simulink library "cooling_system_components"  (R2026a)
settings: Solver=VariableStepAuto
undefined symbols (not defined in the file or in its folder): cooling_system, plate_5p48s_detailled_thr
libraries: fl_lib x14, batt_lib x3, simulink x1, nesl_utility x1
Description:
  | Copyright 2023-2026 The MathWorks, Inc.
settings Model: Creator=smiller  LastModifiedBy=smiller

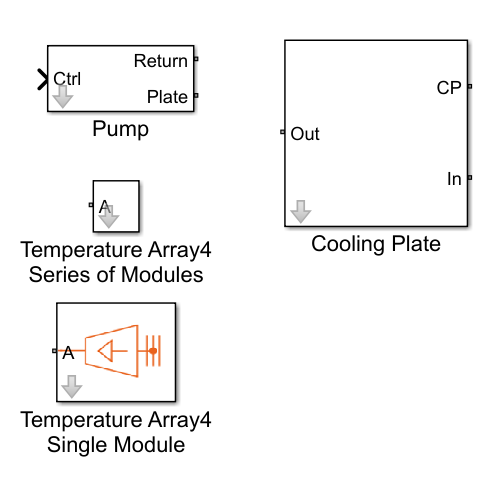
[thumbnail: Simulink's stored preview of the top-level diagram]
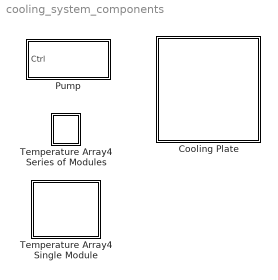
== system cooling_system_components ==
  Cooling Plate : Subsystem  mask{plate=plate_5p48s_detailled_thr}
      mask prompts: plate "Plate Parameters"
  Pump : Subsystem  mask{num_plates=8}
      mask prompts: num_plates "Number of plates"
  Temperature Array4 Series of Modules : Subsystem  mask{ma_num=1, ma_total=8, t_in=16, t_out=23}
      mask prompts: ma_num "Module Assembly Number"; ma_total "Total Module Assemblies"; t_in "Temperature System Inlet (degC)"; t_out "Temperature System Outlet (degC)"
  Temperature Array4 Single Module : Subsystem  mask{t_in=16, t_out=23}
      mask prompts: t_in "Temperature System Inlet (degC)"; t_out "Temperature System Outlet (degC)"
      mask Display: image('ssc_airvtol_cooling_bcs_IMAGE.png');

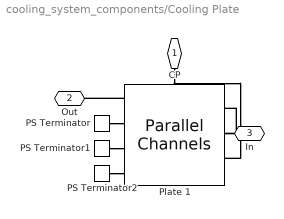
== system cooling_system_components/Cooling Plate ==
  PS Terminator : fl_lib/Physical Signals/Sinks/PS Terminator
  PS Terminator1 : fl_lib/Physical Signals/Sinks/PS Terminator
  PS Terminator2 : fl_lib/Physical Signals/Sinks/PS Terminator
  Plate 1 : batt_lib/Thermal/Parallel Channels  plateConnectivity=simscape.battery.enum.thermal.coolingPlateConnectivity.singleSided  numBattThermalNodes1=plate.Nodes  dimensionThermalNodes1=plate.Dimensions  locationThermalNodes1=plate.Coordinates  numBattThermalNodes2=1  dimensionThermalNodes2=ones(1, 2)  locationThermalNodes2=ones(1, 2)  plateDimX=plate.partitions_x  plateDimY=plate.partitions_y  plateTh=plate.thickness m  plateThCond=plate.k_thermal W/(K*m)  plateDen=plate.rho kg/m^3  plateCp=plate.cp J/(K*kg)  plateTemp_ini=plate.coolant_temp K  Re_lam=2000  Re_tur=4000  Nu_lam=3.66  length_add=1e-3 m  shape_factor=64  nChannels=plate.num_channels  selectChannelOrientation=simscape.battery.enum.thermal.coolingChannelsDirection.alongX  channelDia=plate.diameter_hyd m  distributorDia=plate.diameter_dst m  roughnessPipe=plate.pipe_rough m
  CP : PMIOPort  Side=Left
  Out : PMIOPort  Port=2  Side=Right
  In : PMIOPort  Port=3  Side=Left
  connections:
  PS Terminator2/LConn1 -- Plate 1/RConn4
  Plate 1/RConn1 -- Out/RConn1
  In/RConn1 -- Plate 1/LConn1
  CP/RConn1 -- Plate 1/LConn2
  PS Terminator1/LConn1 -- Plate 1/RConn3
  PS Terminator/LConn1 -- Plate 1/RConn2

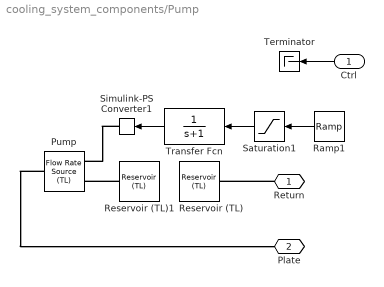
== system cooling_system_components/Pump ==
  Ctrl : Inport
  Pump : fl_lib/Thermal Liquid/Sources/Flow Rate Source (TL)  source_type=foundation.enum.constant_controlled.controlled  flow_type=foundation.enum.mass_volumetric_flow.mass  mass_flow=0 kg/s  volumetric_flow=0 m^3/s  power_spec=foundation.enum.power_spec.isentropic  area=0.01 m^2
  Ramp1 : simulink/Sources/Ramp  slope=cooling_system.on_rate  start=1  InitialOutput=0
  Reservoir (TL) : fl_lib/Thermal Liquid/Elements/Reservoir (TL)  pressure_input=false  pressure_spec=foundation.enum.pressure_spec.atmospheric  reservoir_pressure=0.101325 MPa  temperature_input=false  reservoir_temperature=cooling_system.coolant_temp(2) K  area=0.01 m^2  input_error_spec=foundation.enum.input_range_error.warn
  Reservoir (TL)1 : fl_lib/Thermal Liquid/Elements/Reservoir (TL)  pressure_input=false  pressure_spec=foundation.enum.pressure_spec.atmospheric  reservoir_pressure=0.101325 MPa  temperature_input=false  reservoir_temperature=cooling_system.coolant_temp(1) K  area=0.01 m^2  input_error_spec=foundation.enum.input_range_error.warn
  Saturation1 : Saturate  UpperLimit=cooling_system.pump_max_flow*num_plates  LowerLimit=0  ZeroCross=off
  Simulink-PS Converter1 : nesl_utility/Simulink-PS Converter  PhysicalDomain=network_engine_domain  SubClassName=ps_input  LeftPortType=input  RightPortType=output  PseudoPeriodic=off  Frequencies=[]  NoiseDistribution=none  NoiseParameters=[]  Unit=kg/s  AffineConversion=off  FilteringAndDerivatives=provide  SimscapeFilterOrder=1  InputFilterTimeConstant=0.001  UdotUserProvided=0
  Terminator : Terminator
  Transfer Fcn : TransferFcn  Denominator=[1 1]
  Return : PMIOPort  Side=Right
  Plate : PMIOPort  Port=2  Side=Right
  wires:
  Ctrl/1 -> Terminator/1
  Ramp1/1 -> Saturation1/1
  Saturation1/1 -> Transfer Fcn/1
  Transfer Fcn/1 -> Simulink-PS Converter1/1
  connections:
  Pump/RConn1 -- Plate/RConn1
  Return/RConn1 -- Reservoir (TL)/LConn1
  Reservoir (TL)1/LConn1 -- Pump/LConn1
  Simulink-PS Converter1/RConn1 -- Pump/LConn2

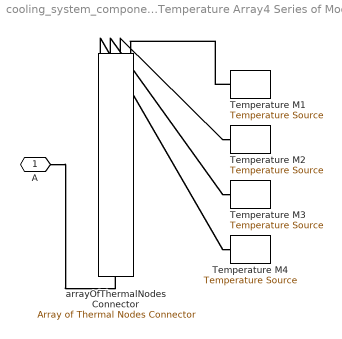
== system cooling_system_components/Temperature Array4 Series of Modules ==
  Temperature M1 : fl_lib/Thermal/Thermal Sources/Temperature Source  temperature=t_in+(t_out-t_in)*(ma_num-1+0/3)/(ma_total-1) degC
  Temperature M2 : fl_lib/Thermal/Thermal Sources/Temperature Source  temperature=t_in+(t_out-t_in)*(ma_num-1+1/3)/(ma_total-1) degC
  Temperature M3 : fl_lib/Thermal/Thermal Sources/Temperature Source  temperature=t_in+(t_out-t_in)*(ma_num-1+2/3)/(ma_total-1) degC
  Temperature M4 : fl_lib/Thermal/Thermal Sources/Temperature Source  temperature=t_in+(t_out-t_in)*(ma_num-1+3/3)/(ma_total-1) degC
  arrayOfThermalNodesConnector : batt_lib/Thermal/Array of Thermal Nodes Connector  numInputConnections=simscape.battery.enum.thermal.numArrayOfNodesConnections.four  concatenateDimension=2  complementaryDimensionsSize=1  inNode1NumElements=1  inNode2NumElements=1  inNode3NumElements=1  inNode4NumElements=1  inNode5NumElements=1  inNode6NumElements=1  inNode7NumElements=1  inNode8NumElements=1  inNode9NumElements=1  inNode10NumElements=1  inNode11NumElements=1  inNode12NumElements=1  inNode13NumElements=1  inNode14NumElements=1  inNode15NumElements=1  inNode16NumElements=1  inNode17NumElements=1  inNode18NumElements=1  inNode19NumElements=1  inNode20NumElements=1  inNode21NumElements=1  inNode22NumElements=1  inNode23NumElements=1  inNode24NumElements=1  inNode25NumElements=1  inNode26NumElements=1  inNode27NumElements=1  inNode28NumElements=1  inNode29NumElements=1  inNode30NumElements=1  inNode31NumElements=1  inNode32NumElements=1  inNode33NumElements=1  inNode34NumElements=1  inNode35NumElements=1  inNode36NumElements=1  inNode37NumElements=1  inNode38NumElements=1  inNode39NumElements=1  inNode40NumElements=1  inNode41NumElements=1  inNode42NumElements=1  inNode43NumElements=1  inNode44NumElements=1  inNode45NumElements=1  inNode46NumElements=1  inNode47NumElements=1  inNode48NumElements=1  inNode49NumElements=1  inNode50NumElements=1
  A : PMIOPort  Side=Left
  connections:
  A/RConn1 -- arrayOfThermalNodesConnector/RConn1
  Temperature M1/LConn1 -- arrayOfThermalNodesConnector/LConn1
  arrayOfThermalNodesConnector/LConn2 -- Temperature M2/LConn1
  arrayOfThermalNodesConnector/LConn3 -- Temperature M3/LConn1
  arrayOfThermalNodesConnector/LConn4 -- Temperature M4/LConn1

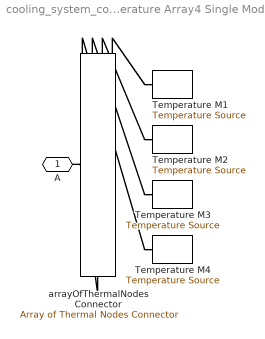
== system cooling_system_components/Temperature Array4 Single Module ==
  Temperature M1 : fl_lib/Thermal/Thermal Sources/Temperature Source  temperature=t_in+(t_out-t_in)*(0/3) degC
  Temperature M2 : fl_lib/Thermal/Thermal Sources/Temperature Source  temperature=t_in+(t_out-t_in)*(1/3) degC
  Temperature M3 : fl_lib/Thermal/Thermal Sources/Temperature Source  temperature=t_in+(t_out-t_in)*(2/3) degC
  Temperature M4 : fl_lib/Thermal/Thermal Sources/Temperature Source  temperature=t_in+(t_out-t_in)*(3/3) degC
  arrayOfThermalNodesConnector : batt_lib/Thermal/Array of Thermal Nodes Connector  numInputConnections=simscape.battery.enum.thermal.numArrayOfNodesConnections.four  concatenateDimension=2  complementaryDimensionsSize=1  inNode1NumElements=1  inNode2NumElements=1  inNode3NumElements=1  inNode4NumElements=1  inNode5NumElements=1  inNode6NumElements=1  inNode7NumElements=1  inNode8NumElements=1  inNode9NumElements=1  inNode10NumElements=1  inNode11NumElements=1  inNode12NumElements=1  inNode13NumElements=1  inNode14NumElements=1  inNode15NumElements=1  inNode16NumElements=1  inNode17NumElements=1  inNode18NumElements=1  inNode19NumElements=1  inNode20NumElements=1  inNode21NumElements=1  inNode22NumElements=1  inNode23NumElements=1  inNode24NumElements=1  inNode25NumElements=1  inNode26NumElements=1  inNode27NumElements=1  inNode28NumElements=1  inNode29NumElements=1  inNode30NumElements=1  inNode31NumElements=1  inNode32NumElements=1  inNode33NumElements=1  inNode34NumElements=1  inNode35NumElements=1  inNode36NumElements=1  inNode37NumElements=1  inNode38NumElements=1  inNode39NumElements=1  inNode40NumElements=1  inNode41NumElements=1  inNode42NumElements=1  inNode43NumElements=1  inNode44NumElements=1  inNode45NumElements=1  inNode46NumElements=1  inNode47NumElements=1  inNode48NumElements=1  inNode49NumElements=1  inNode50NumElements=1
  A : PMIOPort  Side=Left
  connections:
  arrayOfThermalNodesConnector/LConn4 -- Temperature M4/LConn1
  arrayOfThermalNodesConnector/LConn3 -- Temperature M3/LConn1
  arrayOfThermalNodesConnector/LConn2 -- Temperature M2/LConn1
  arrayOfThermalNodesConnector/LConn1 -- Temperature M1/LConn1
  arrayOfThermalNodesConnector/RConn1 -- A/RConn1
